simulink model "Wiper"  (R2023b)
settings: Solver=FixedStepDiscrete  StartTime=0.0  StopTime=10.0  FixedStep=0.01  RelTol=1e-3
libraries: simulink x1
settings Model: ExtModeTrigDuration=2  Creator=Beshary  LastModifiedBy=Beshary
settings OptimizationCC: DefaultParameterBehavior=Inlined  UseDivisionForNetSlopeComputation=on  GainParamInheritBuiltInType=on  UseFloatMulNetSlope=on  InlineInvariantSignals=on  PassReuseOutputArgsAs=Individual arguments  ZeroExternalMemoryAtStartup=off  ZeroInternalMemoryAtStartup=off  NoFixptDivByZeroProtection=on  EfficientFloat2IntCast=on  LifeSpan=1  MaxStackSize=64  OptimizeBlockOrder=speed  DifferentSizesBufferReuse=on  EfficientTunableParamExpr=on
settings DebuggingCC: ParameterTunabilityLossMsg=error
settings HardwareCC: ProdBitPerInt=16  ProdBitPerPointer=16  ProdBitPerSizeT=16  ProdBitPerPtrDiffT=16  ProdLargestAtomicFloat=None  ProdWordSize=8  ProdLongLongMode=on  ProdHWDeviceType=Atmel->AVR
settings SFSimCC: MATLABDynamicMemAlloc=off
settings RTWCC: Description=Embedded Coder  SystemTargetFile=ert.tlc  HardwareBoard=Arduino Uno  TemplateMakefile=ert_default_tmf  Toolchain=Arduino AVR  BuildConfiguration=Faster Runs
settings CodeAppCC: ForceParamTrailComments=on  IgnoreCustomStorageClasses=off  OperatorAnnotations=on  SimulinkDataObjDesc=on  SFDataObjDesc=on  CustomSymbolStrGlobalVar=rt$N$M  CustomSymbolStrType=$N$M  CustomSymbolStrFcn=$N$M$F  CustomSymbolStrMacro=$N$M  InsertBlockDesc=on
settings ERTTargetCC: IncludeMdlTerminateFcn=off  CombineSignalStateStructs=on  SuppressErrorStatus=on  SupportAbsoluteTime=off  SupportComplex=off  ExtModeTransport=3  ExtModeStaticAlloc=on  ExtModeAutomaticAllocSize=off  ExtModeStaticAllocSize=250  ExtModeMexFile=ext_xcp  ExtModeIntrfLevel=Level2 - Open  InlinedParameterPlacement=NonHierarchical  ERTFilePackagingFormat=CompactWithDataFile

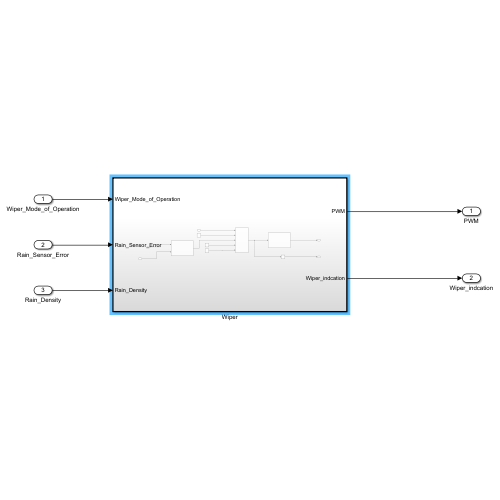
[thumbnail: Simulink's stored preview of the top-level diagram]
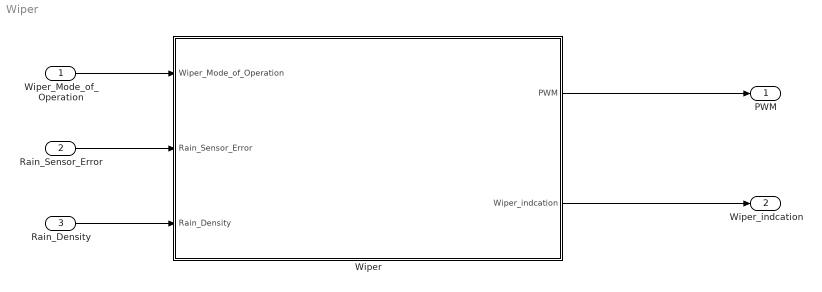
== system Wiper ==
  Wiper_Mode_of_Operation : Inport  OutDataTypeStr=Enum: Operation_Mode
  Rain_Sensor_Error : Inport  Port=2
  Rain_Density : Inport  Port=3
  Wiper : Subsystem  TreatAsAtomicUnit=on
  PWM : Outport
  Wiper_indcation : Outport  Port=2
  wires:
  Wiper_Mode_of_Operation/1 -> Wiper/1(Wiper_Mode_of_Operation)
  Rain_Sensor_Error/1 -> Wiper/2(Rain_Sensor_Error)
  Rain_Density/1 -> Wiper/3(Rain_Density)
  Wiper/1(PWM) -> PWM/1
  Wiper/2(Wiper_indcation) -> Wiper_indcation/1

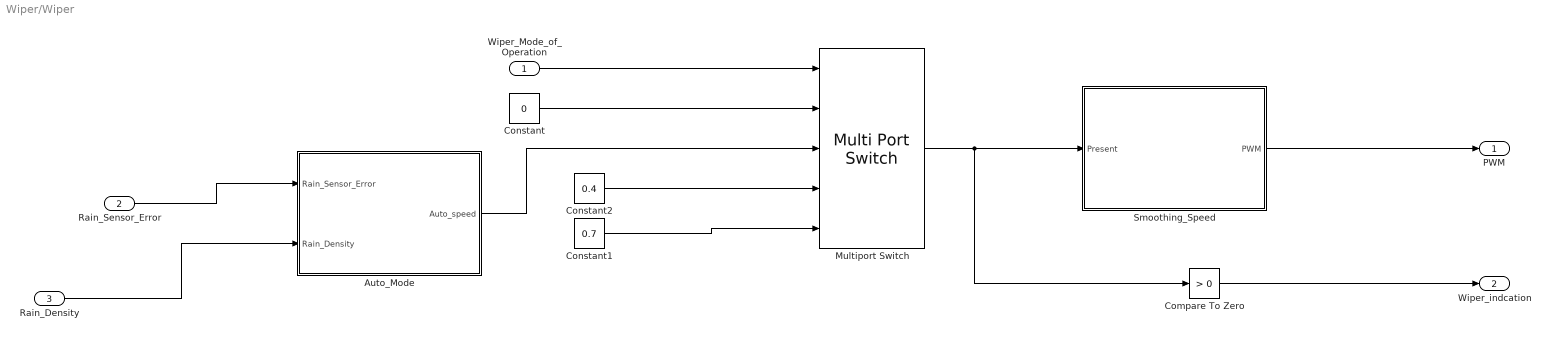
== system Wiper/Wiper ==
  Wiper_Mode_of_Operation : Inport
  Rain_Sensor_Error : Inport  Port=2
  Rain_Density : Inport  Port=3
  Auto_Mode : Subsystem
  Compare To Zero : simulink/Logic and Bit Operations/Compare To Zero  relop=>  OutDataTypeStr=boolean
  Constant : Constant  Value=0
  Constant1 : Constant  Value=0.7
  Constant2 : Constant  Value=0.4
  Multiport Switch : MultiPortSwitch  DataPortOrder=Specify indices  DataPortIndices={Operation_Mode.OFF,Operation_Mode.Auto,Operation_Mode.Low_Speed,Operation_Mode.High_Speed}  DiagnosticForDefault=None  SaturateOnIntegerOverflow=off  InputSameDT=off
  Smoothing_Speed : Subsystem
  PWM : Outport
  Wiper_indcation : Outport  Port=2
  wires:
  Wiper_Mode_of_Operation/1 -> Multiport Switch/1
  Constant/1 -> Multiport Switch/2
  Constant2/1 -> Multiport Switch/4
  Constant1/1 -> Multiport Switch/5
  Rain_Sensor_Error/1 -> Auto_Mode/1(Rain_Sensor_Error)
  Rain_Density/1 -> Auto_Mode/2(Rain_Density)
  Auto_Mode/1(Auto_speed) -> Multiport Switch/3
  Multiport Switch/1 -> Compare To Zero/1, Smoothing_Speed/1(Present)
  Smoothing_Speed/1(PWM) -> PWM/1
  Compare To Zero/1 -> Wiper_indcation/1

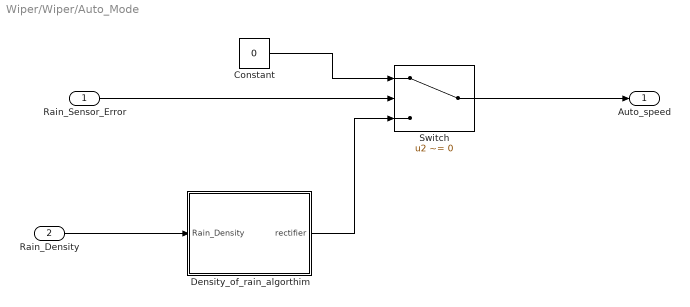
== system Wiper/Wiper/Auto_Mode ==
  Rain_Sensor_Error : Inport
  Rain_Density : Inport  Port=2
  Constant : Constant  Value=0
  Density_of_rain_algorthim : Subsystem
  Switch : Switch  Criteria=u2 ~= 0  SaturateOnIntegerOverflow=off  InputSameDT=off
  Auto_speed : Outport
  wires:
  Rain_Sensor_Error/1 -> Switch/2
  Constant/1 -> Switch/1
  Rain_Density/1 -> Density_of_rain_algorthim/1(Rain_Density)
  Density_of_rain_algorthim/1(rectifier) -> Switch/3
  Switch/1 -> Auto_speed/1

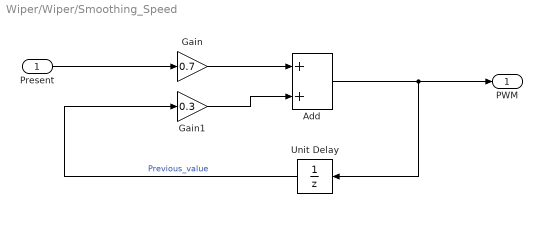
== system Wiper/Wiper/Smoothing_Speed ==
  Present : Inport
  Add : Sum
  Gain : Gain  Gain=0.7
  Gain1 : Gain  Gain=0.3
  Unit Delay : UnitDelay  SampleTime=-1  HasFrameUpgradeWarning=on
  PWM : Outport
  wires:
  Gain/1 -> Add/1
  Present/1 -> Gain/1
  Unit Delay/1 -> Gain1/1  "Previous_value"
  Gain1/1 -> Add/2
  Add/1 -> Unit Delay/1, PWM/1

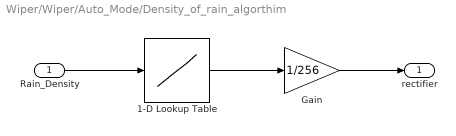
== system Wiper/Wiper/Auto_Mode/Density_of_rain_algorthim ==
  Rain_Density : Inport
  1-D Lookup Table : Lookup_n-D  NumberOfTableDimensions=1  BreakpointsForDimension1=[0 256 512 768 1023]  Table=[0 64 128 192 256]  InternalRulePriority=Speed  RndMeth=Simplest
  Gain : Gain  Gain=1/256
  rectifier : Outport
  wires:
  1-D Lookup Table/1 -> Gain/1
  Gain/1 -> rectifier/1
  Rain_Density/1 -> 1-D Lookup Table/1
